simulink model "BASELINE_PARTITION"  (R2019b)
settings: Solver=VariableStepAuto  StartTime=0.0  StopTime=10.0  RelTol=1e-3
undefined symbols (not defined in the file): baseline_force, Dt, max_force_1N, max_force_1P, V_nom, x_lut_1N, x_lut_1P, x_table_0N, x_table_0P, y_lut_1N, y_lut_1P, y_table_0N, y_table_0P
settings Model: Creator=peter  LastModifiedBy=peter

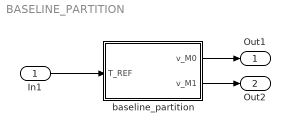
== system BASELINE_PARTITION ==
  In1 : Inport
  baseline_partition : Subsystem
  Out1 : Outport
  Out2 : Outport  Port=2
  wires:
  In1/1 -> baseline_partition/1("T_REF ")
  baseline_partition/1("v_M0 ") -> Out1/1
  baseline_partition/2("v_M1 ") -> Out2/1

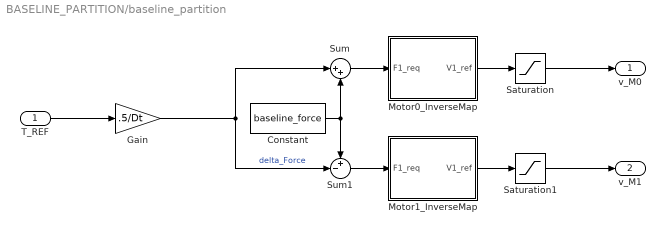
== system BASELINE_PARTITION/baseline_partition ==
  "T_REF " : Inport
  Constant : Constant  Value=baseline_force
  Gain : Gain  Gain=.5/Dt
  Motor0_InverseMap : Subsystem
  Motor1_InverseMap : Subsystem
  Saturation : Saturate  UpperLimit=V_nom  LowerLimit=-V_nom
  Saturation1 : Saturate  UpperLimit=V_nom  LowerLimit=-V_nom
  Sum : Sum  Inputs=|++
  Sum1 : Sum  Inputs=+-|
  "v_M0 " : Outport
  "v_M1 " : Outport  Port=2
  wires:
  "T_REF "/1 -> Gain/1
  Gain/1 -> Sum/1, Sum1/2  "delta_Force"
  Motor0_InverseMap/1(V1_ref) -> Saturation/1
  Motor1_InverseMap/1(V1_ref) -> Saturation1/1
  Sum/1 -> Motor0_InverseMap/1(F1_req)
  Sum1/1 -> Motor1_InverseMap/1(F1_req)
  Constant/1 -> Sum1/1, Sum/2
  Saturation1/1 -> "v_M1 "/1
  Saturation/1 -> "v_M0 "/1

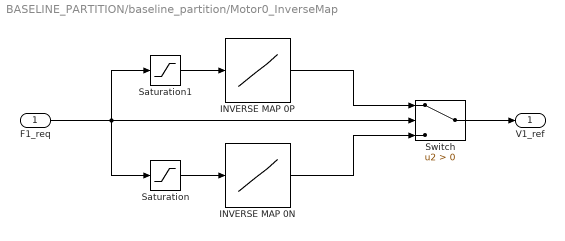
== system BASELINE_PARTITION/baseline_partition/Motor0_InverseMap ==
  F1_req : Inport
  INVERSE MAP 0N : Lookup_n-D  NumberOfTableDimensions=1  LookupTableObject=gigi  BreakpointsForDimension1=x_table_0N  BeginIndexSearchUsingPreviousIndexResult=on  Table=y_table_0N  DiagnosticForOutOfRangeInput=Warning  InternalRulePriority=Speed  RndMeth=Simplest  InputSameDT=on
  INVERSE MAP 0P : Lookup_n-D  NumberOfTableDimensions=1  LookupTableObject=gigi  BreakpointsForDimension1=x_table_0P  BeginIndexSearchUsingPreviousIndexResult=on  Table=y_table_0P  DiagnosticForOutOfRangeInput=Warning  InternalRulePriority=Speed  RndMeth=Simplest  InputSameDT=on
  Saturation : Saturate  UpperLimit=0  LowerLimit=max_force_1N
  Saturation1 : Saturate  UpperLimit=max_force_1P  LowerLimit=0
  Switch : Switch  Criteria=u2 > Threshold
  V1_ref : Outport
  wires:
  Saturation1/1 -> INVERSE MAP 0P/1
  F1_req/1 -> Saturation/1, Switch/2, Saturation1/1
  Saturation/1 -> INVERSE MAP 0N/1
  Switch/1 -> V1_ref/1
  INVERSE MAP 0P/1 -> Switch/1
  INVERSE MAP 0N/1 -> Switch/3

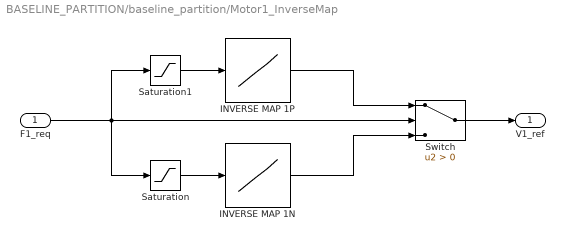
== system BASELINE_PARTITION/baseline_partition/Motor1_InverseMap ==
  F1_req : Inport
  INVERSE MAP 1N : Lookup_n-D  NumberOfTableDimensions=1  LookupTableObject=gigi  BreakpointsForDimension1=x_lut_1N  BeginIndexSearchUsingPreviousIndexResult=on  Table=y_lut_1N  DiagnosticForOutOfRangeInput=Warning  InternalRulePriority=Speed  RndMeth=Simplest  InputSameDT=on
  INVERSE MAP 1P : Lookup_n-D  NumberOfTableDimensions=1  LookupTableObject=gigi  BreakpointsForDimension1=x_lut_1P  BeginIndexSearchUsingPreviousIndexResult=on  Table=y_lut_1P  DiagnosticForOutOfRangeInput=Warning  InternalRulePriority=Speed  RndMeth=Simplest  InputSameDT=on
  Saturation : Saturate  UpperLimit=0  LowerLimit=max_force_1N
  Saturation1 : Saturate  UpperLimit=max_force_1P  LowerLimit=0
  Switch : Switch  Criteria=u2 > Threshold
  V1_ref : Outport
  wires:
  Saturation1/1 -> INVERSE MAP 1P/1
  F1_req/1 -> Saturation/1, Switch/2, Saturation1/1
  Saturation/1 -> INVERSE MAP 1N/1
  Switch/1 -> V1_ref/1
  INVERSE MAP 1P/1 -> Switch/1
  INVERSE MAP 1N/1 -> Switch/3
